simulink model "Simulation"  (R2026a)
settings: Solver=VariableStepAuto
settings DataIOCC: TimeSaveName=t
settings DebuggingCC: ArtificialAlgebraicLoopMsg=none  MaxConsecutiveZCsMsg=none

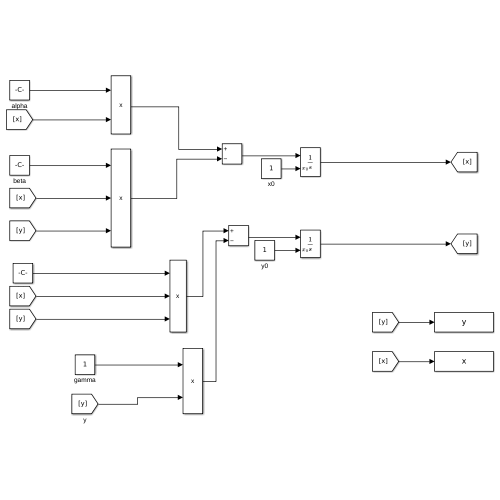
[thumbnail: Simulink's stored preview of the top-level diagram]
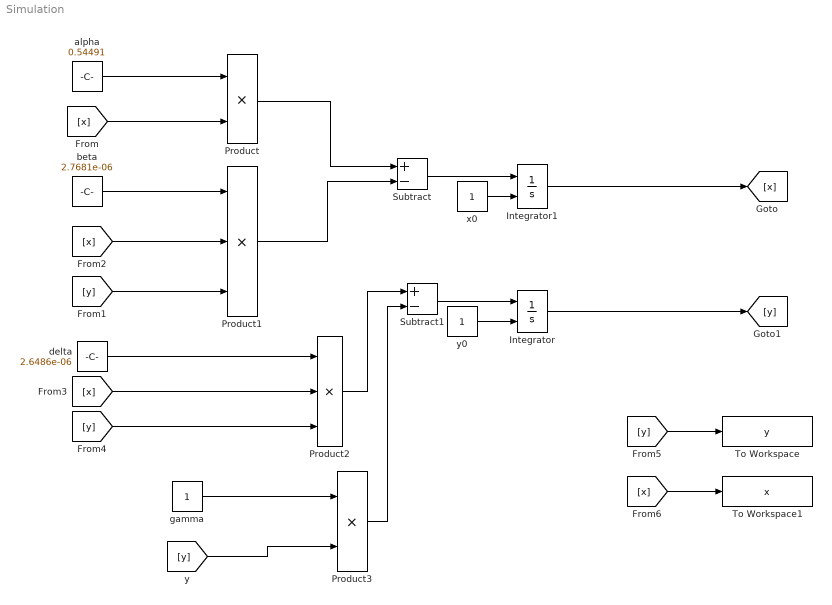
== system Simulation ==
  Integrator : Integrator  InitialConditionSource=external
  Integrator1 : Integrator  InitialConditionSource=external
  Product : Product
  Product1 : Product  Inputs=3
  Product2 : Product  Inputs=3
  Product3 : Product
  Subtract : Sum  Inputs=+-
  Subtract1 : Sum  Inputs=+-
  To Workspace : ToWorkspace  VariableName=y  SampleTime=-1
  To Workspace1 : ToWorkspace  VariableName=x  SampleTime=-1
  alpha : Constant  Value=0.54491
  beta : Constant  Value=2.7681e-06
  delta : Constant  Value=2.6486e-06
  gamma : Constant
  x0 : Constant
  y0 : Constant
  wires:
  Integrator1/1 -> [x]
  Integrator/1 -> [y]
  y0/1 -> Integrator/2
  x0/1 -> Integrator1/2
  Subtract/1 -> Integrator1/1
  Subtract1/1 -> Integrator/1
  Product/1 -> Subtract/1
  Product1/1 -> Subtract/2
  alpha/1 -> Product/1
  [x] -> Product/2
  [x] -> Product1/2
  Product2/1 -> Subtract1/1
  Product3/1 -> Subtract1/2
  delta/1 -> Product2/1
  [x] -> Product2/2
  [y] -> Product2/3
  [y] -> To Workspace/1
  [x] -> To Workspace1/1
  beta/1 -> Product1/1
  [y] -> Product1/3
  gamma/1 -> Product3/1
  [y] -> Product3/2
